simulink subsystem "YawController_SubSystem"  (R2020b)
settings: Solver=VariableStepAuto  StartTime=0.0  StopTime=10.0  RelTol=1e-3
undefined symbols (not defined in the file): DiscIntNeverNeededParam, drv, Ts, yaw_Ki, yaw_Kp
settings Model: Creator=utente-A  LastModifiedBy=Musta
settings DebuggingCC: SFMachineParentedDataDiag=error

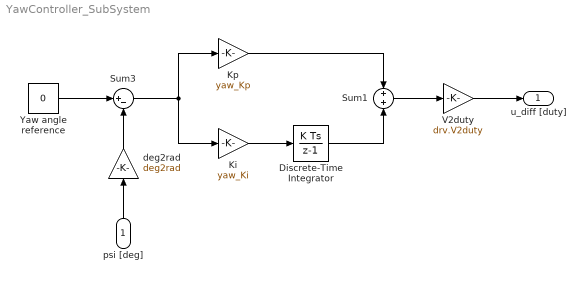
== system YawController_SubSystem ==
  psi [deg] : Inport
  Discrete-Time Integrator : DiscreteIntegrator  SampleTime=Ts  ICPrevOutput=DiscIntNeverNeededParam  ICPrevScaledInput=DiscIntNeverNeededParam
  Ki : Gain  Gain=yaw_Ki
  Kp : Gain  Gain=yaw_Kp
  Sum1 : Sum
  Sum3 : Sum  Inputs=|+-
  V2duty : Gain  Gain=drv.V2duty
  Yaw angle reference : Constant  Value=0
  deg2rad : Gain  Gain=deg2rad
  u_diff [duty] : Outport
  wires:
  Sum3/1 -> Kp/1, Ki/1
  psi [deg]/1 -> deg2rad/1
  deg2rad/1 -> Sum3/2
  Ki/1 -> Discrete-Time Integrator/1
  Kp/1 -> Sum1/1
  Discrete-Time Integrator/1 -> Sum1/2
  Sum1/1 -> V2duty/1
  V2duty/1 -> u_diff [duty]/1
  Yaw angle reference/1 -> Sum3/1
